simulink subsystem "rss_SysSTM_CRRC"  (R2023a)
settings: Solver=VariableStepAuto  StartTime=0.0  StopTime=10.0  RelTol=1e-3
undefined symbols (not defined in the file): Cdbl_nElecAgSpdMaxVal, Gs16_nShOffActElecSpd_C, Gu16_ctSysStInitWaitCnt_C
settings Model: Creator=xiaoqiang.yuan  LastModifiedBy=xiaoqiang.yuan

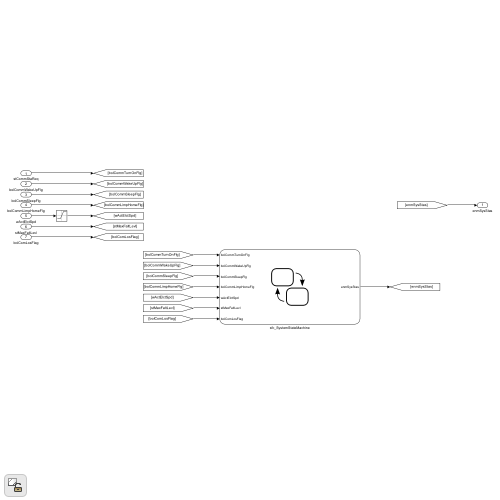
[thumbnail: Simulink's stored preview of the top-level diagram]
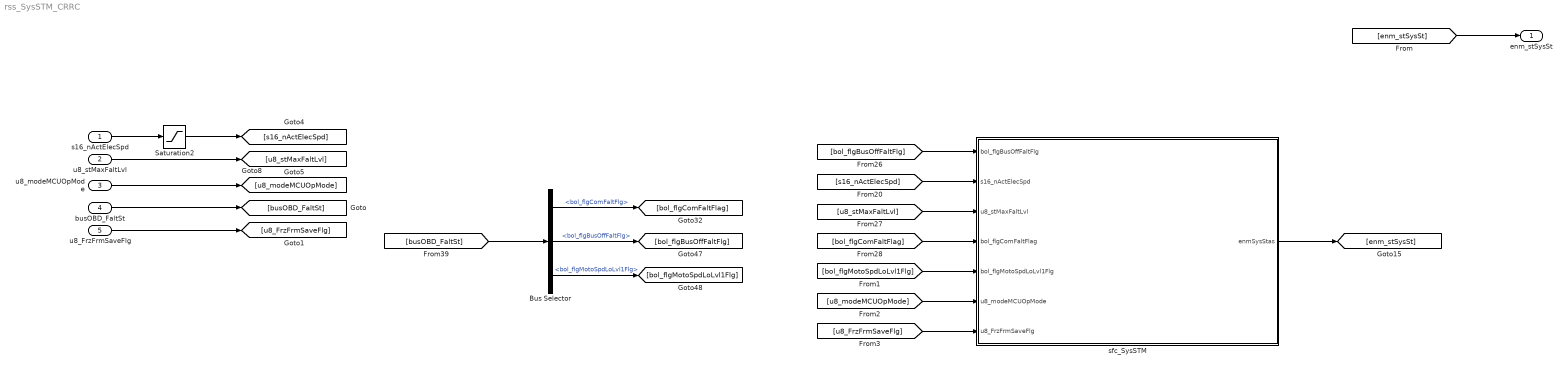
== system rss_SysSTM_CRRC ==
  s16_nActElecSpd : Inport  OutDataTypeStr=dt_Standardize_s16p15b0
  u8_stMaxFaltLvl : Inport  Port=2  OutDataTypeStr=uint8
  u8_modeMCUOpMode : Inport  Port=3  OutDataTypeStr=uint8
  busOBD_FaltSt : Inport  Port=4  OutDataTypeStr=Bus: BUS_OBD_FALT_STS
  u8_FrzFrmSaveFlg : Inport  Port=5  OutDataTypeStr=uint8
  Bus Selector : BusSelector  OutputSignals=bol_flgComFaltFlg,bol_flgBusOffFaltFlg,bol_flgMotoSpdLoLvl1Flg
  Saturation2 : Saturate  UpperLimit=Cdbl_nElecAgSpdMaxVal  LowerLimit=-Cdbl_nElecAgSpdMaxVal
  sfc_SysSTM : Stateflow chart  TreatAsAtomicUnit=on
  enm_stSysSt : Outport  OutDataTypeStr=Enum: ENM_SYS_STATUS
  wires:
  [bol_flgBusOffFaltFlg] -> sfc_SysSTM/1(bol_flgBusOffFaltFlg)
  [s16_nActElecSpd] -> sfc_SysSTM/2(s16_nActElecSpd)
  [u8_stMaxFaltLvl] -> sfc_SysSTM/3(u8_stMaxFaltLvl)
  [bol_flgComFaltFlag] -> sfc_SysSTM/4(bol_flgComFaltFlag)
  u8_stMaxFaltLvl/1 -> [u8_stMaxFaltLvl]
  s16_nActElecSpd/1 -> Saturation2/1
  [enm_stSysSt] -> enm_stSysSt/1
  sfc_SysSTM/1(enmSysStas) -> [enm_stSysSt]
  Saturation2/1 -> [s16_nActElecSpd]
  [bol_flgMotoSpdLoLvl1Flg] -> sfc_SysSTM/5(bol_flgMotoSpdLoLvl1Flg)
  u8_modeMCUOpMode/1 -> [u8_modeMCUOpMode]
  [u8_modeMCUOpMode] -> sfc_SysSTM/6(u8_modeMCUOpMode)
  [busOBD_FaltSt] -> Bus Selector/1
  busOBD_FaltSt/1 -> [busOBD_FaltSt]
  Bus Selector/1 -> [bol_flgComFaltFlag]  "<bol_flgComFaltFlg>"
  Bus Selector/2 -> [bol_flgBusOffFaltFlg]  "<bol_flgBusOffFaltFlg>"
  Bus Selector/3 -> [bol_flgMotoSpdLoLvl1Flg]  "<bol_flgMotoSpdLoLvl1Flg>"
  u8_FrzFrmSaveFlg/1 -> [u8_FrzFrmSaveFlg]
  [u8_FrzFrmSaveFlg] -> sfc_SysSTM/7(u8_FrzFrmSaveFlg)

== stateflow chart rss_SysSTM_CRRC/sfc_SysSTM ==
  state SYSINIT
    en:
    enmSysStas = ENM_SYS_STATUS.SYSINIT;
    u16_ctSysStInitWaitCnt = uint16(0);
    du:
    u16_ctSysStInitWaitCnt = u16_ctSysStInitWaitCnt + uint16(1);
    ex:
    u16_ctSysStInitWaitCnt = uint16(0);
  state NORMAL
    state STANDBY
      en:
      enmSysStas = ENM_SYS_STATUS.STANDBY;
    state RUN
      en:
      enmSysStas = ENM_SYS_STATUS.RUN;
    state SYSDERATING
      en:
      enmSysStas = ENM_SYS_STATUS.SYSDERATING;
    (default) -> STANDBY
    STANDBY -> RUN : [u8_modeMCUOpMode ==uint8(1)]
    RUN -> STANDBY [order 1] : [u8_modeMCUOpMode ==uint8(3)]
    RUN -> SYSDERATING [order 2] : [bol_flgMotoSpdLoLvl1Flg]
    SYSDERATING -> RUN : [~bol_flgMotoSpdLoLvl1Flg]
  state SYSFAIL
    en:
    enmSysStas = ENM_SYS_STATUS.SYSFAIL;
  state LIMPHOME
    en:
    enmSysStas = ENM_SYS_STATUS.LIMPHOME;
  state SYSSLEEP
    en:
    enmSysStas = ENM_SYS_STATUS.SYSSLEEP;
  (default) -> SYSINIT
  SYSINIT -> NORMAL : [u16_ctSysStInitWaitCnt >= Gu16_ctSysStInitWaitCnt_C &&...
      | u8_modeMCUOpMode ==uint8(0)]
  NORMAL -> SYSFAIL [order 1] : [u8_stMaxFaltLvl ==uint8(3)]
  LIMPHOME -> SYSFAIL [order 1] : [u8_stMaxFaltLvl ==uint8(3)]
  SYSFAIL -> NORMAL [order 1] : [u8_stMaxFaltLvl ~=uint8(3)]
  SYSFAIL -> (junction 142) [order 2] : [u8_modeMCUOpMode ==uint8(2) &&...
      | abs(s16_nActElecSpd) < abs(Gs16_nShOffActElecSpd_C) &&...
      | u8_FrzFrmSaveFlg == uint8(1)]
  NORMAL -> LIMPHOME [order 2] : [bol_flgBusOffFaltFlg ||...
      | bol_flgComFaltFlag]
  LIMPHOME -> NORMAL [order 2] : [~bol_flgBusOffFaltFlg &&...
      | ~bol_flgComFaltFlag]
  LIMPHOME -> (junction 140) [order 3] : [u8_modeMCUOpMode ==uint8(2) &&...
      | abs(s16_nActElecSpd) < abs(Gs16_nShOffActElecSpd_C) &&...
      | u8_FrzFrmSaveFlg == uint8(1)]
  NORMAL -> (junction 145) [order 3] : [u8_modeMCUOpMode ==uint8(2) &&...
      | abs(s16_nActElecSpd) < abs(Gs16_nShOffActElecSpd_C) &&...
      | u8_FrzFrmSaveFlg == uint8(1)]
  (junction 140) -> (junction 142)
  (junction 142) -> (junction 145)
  (junction 145) -> SYSSLEEP
  data: bol_flgBusOffFaltFlg input boolean; s16_nActElecSpd input dt_Standardize_s16p15b0; u8_stMaxFaltLvl input uint8; enmSysStas output Enum: ENM_SYS_STATUS; u16_ctSysStInitWaitCnt local uint16; bol_flgComFaltFlag input boolean; Gs16_nShOffActElecSpd_C parameter; Gu16_ctSysStInitWaitCnt_C parameter; bol_flgMotoSpdLoLvl1Flg input boolean; u8_modeMCUOpMode input uint8; u8_FrzFrmSaveFlg input uint8
